simulink model "estymacja_obiekt2_18a"  (R2018a)
settings: Solver=FixedStepDiscrete  StartTime=0.0  StopTime=10.0  FixedStep=0.1  RelTol=1e-3
libraries: sharedTrackingLibrary x1
settings Model: Creator=Dominik  LastModifiedBy=a.kuligowski
settings CodeAppCC: StateflowObjectComments=on

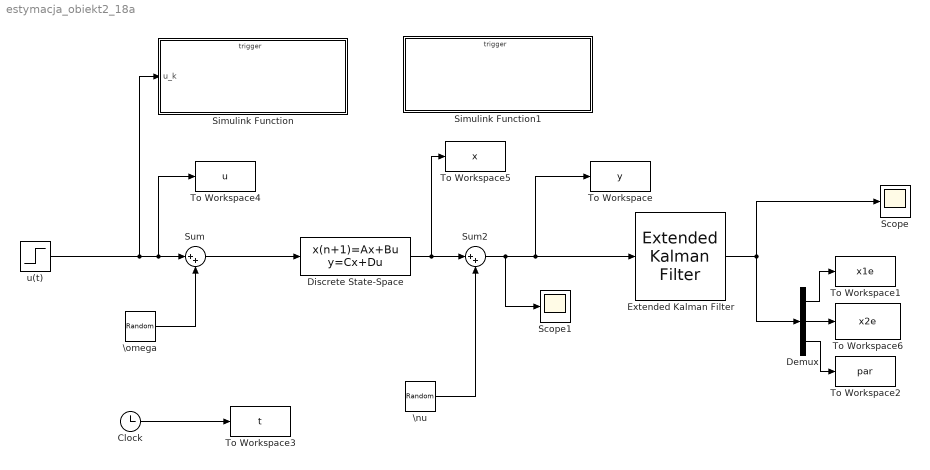
== system estymacja_obiekt2_18a ==
  Clock : Clock
  Demux : Demux  Outputs=3
  Discrete State-Space : DiscreteStateSpace  A=[0.99 0.095; -0.19 0.9]  B=[0.005; 0.095]  C=[1 0]  D=0  InitialCondition=[0;0]  SampleTime=0.1
  Extended Kalman Filter : sharedTrackingLibrary/Extended Kalman Filter  StateTransitionFcn=myStateTransitionFcn  HasStateTransitionJacobianFcn=off  HasAdditiveProcessNoise=Additive  ProcessNoise=diag([0.0005 0.0005 0.0005])  HasTimeVaryingProcessNoise=off  HasStateTransitionFcnExtraArgument=0  InitialState=[0 0 0.2]  InitialStateCovariance=1  MeasurementFcn1=myMeasurementFcn  HasMeasurementJacobianFcn1=off  HasMeasurementEnablePort1=off  HasAdditiveMeasurementNoise1=Additive  MeasurementNoise1=0.0001  HasTimeVaryingMeasurementNoise1=off  HasMeasurementFcnExtraArgument1=0  MeasurementFcn2=myMeasurementFcn  HasMeasurementJacobianFcn2=off  HasMeasurementEnablePort2=off  HasAdditiveMeasurementNoise2=Additive  MeasurementNoise2=1  HasTimeVaryingMeasurementNoise2=off  HasMeasurementFcnExtraArgument2=0  MeasurementFcn3=myMeasurementFcn  HasMeasurementJacobianFcn3=off  HasMeasurementEnablePort3=off  HasAdditiveMeasurementNoise3=Additive  MeasurementNoise3=1  HasTimeVaryingMeasurementNoise3=off  HasMeasurementFcnExtraArgument3=0  MeasurementFcn4=myMeasurementFcn  HasMeasurementJacobianFcn4=off  HasMeasurementEnablePort4=off  HasAdditiveMeasurementNoise4=Additive  MeasurementNoise4=1  HasTimeVaryingMeasurementNoise4=off  HasMeasurementFcnExtraArgument4=0  MeasurementFcn5=myMeasurementFcn  HasMeasurementJacobianFcn5=off  HasMeasurementEnablePort5=off  HasAdditiveMeasurementNoise5=Additive  MeasurementNoise5=1  HasTimeVaryingMeasurementNoise5=off  HasMeasurementFcnExtraArgument5=0  EnableMultirate=off  StateTransitionFcnSampleTime=1  MeasurementFcn1SampleTime=1  MeasurementFcn2SampleTime=1  MeasurementFcn3SampleTime=1  MeasurementFcn4SampleTime=1  MeasurementFcn5SampleTime=1  UseCurrentEstimator=on  OutputStateCovariance=off  DataType=double  SampleTime=0.1  NumberOfMeasurements=1
      settings: SourceProductName=Control System Toolbox  SourceProductBaseCode=CT
  Scope : Scope
  Scope1 : Scope
  Simulink Function : Subsystem  TreatAsAtomicUnit=on
  Simulink Function1 : Subsystem  TreatAsAtomicUnit=on
  Sum : Sum  Inputs=|++
  Sum2 : Sum  Inputs=|++
  To Workspace : ToWorkspace  VariableName=y  SampleTime=-1
  To Workspace1 : ToWorkspace  VariableName=x1e  SampleTime=-1
  To Workspace2 : ToWorkspace  VariableName=par  SampleTime=-1
  To Workspace3 : ToWorkspace  VariableName=t  SampleTime=-1
  To Workspace4 : ToWorkspace  VariableName=u  SampleTime=-1
  To Workspace5 : ToWorkspace  VariableName=x  SampleTime=-1
  To Workspace6 : ToWorkspace  VariableName=x2e  SampleTime=-1
  \nu : RandomNumber  Variance=0  Seed=11  SampleTime=0.1
  \omega : RandomNumber  Variance=0.0005  Seed=21  SampleTime=0.1
  u(t) : Step  SampleTime=0
  wires:
  Extended Kalman Filter/1 -> Demux/1, Scope/1
  Discrete State-Space/1 -> To Workspace5/1, Sum2/1
  Sum2/1 -> Scope1/1, To Workspace/1, Extended Kalman Filter/1
  \omega/1 -> Sum/2
  \nu/1 -> Sum2/2
  u(t)/1 -> Simulink Function/1(u_k), To Workspace4/1, Sum/1
  Demux/3 -> To Workspace2/1
  Demux/1 -> To Workspace1/1
  Clock/1 -> To Workspace3/1
  Sum/1 -> Discrete State-Space/1
  Demux/2 -> To Workspace6/1

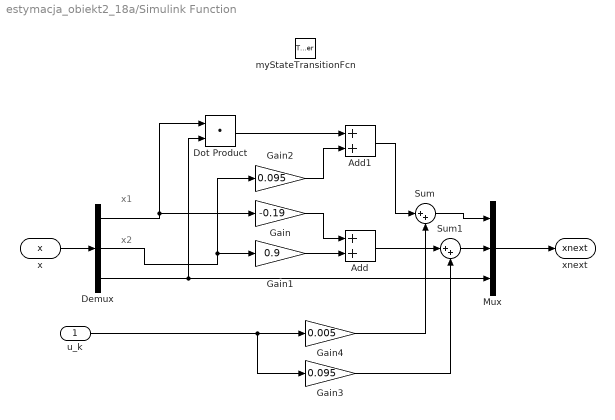
== system estymacja_obiekt2_18a/Simulink Function ==
  note: x2
  note: x1
  u_k : Inport
  myStateTransitionFcn : TriggerPort  TriggerType=function-call  IsSimulinkFunction=on  FunctionName=myStateTransitionFcn  VariantControl=Variant
  Add : Sum
  Add1 : Sum
  Demux : Demux  Outputs=3
  Dot Product : DotProduct  InputSameDT=on  OutDataTypeStr=Inherit: Inherit via internal rule
  Gain : Gain  Gain=-0.19
  Gain1 : Gain  Gain=0.9
  Gain2 : Gain  Gain=0.095
  Gain3 : Gain  Gain=0.095
  Gain4 : Gain  Gain=0.005
  Mux : Mux  Inputs=3
  Sum : Sum  Inputs=|++
  Sum1 : Sum  Inputs=|++
  x : ArgIn  DisableCoverage=on  PortDimensions=3  ArgumentName=x
  xnext : ArgOut  DisableCoverage=on  PortDimensions=3  ArgumentName=xnext
  wires:
  x/1 -> Demux/1
  Demux/3 -> Mux/3, Dot Product/2
  Dot Product/1 -> Add1/1
  Demux/1 -> Dot Product/1, Gain/1
  Sum/1 -> Mux/1
  Mux/1 -> xnext/1
  u_k/1 -> Gain3/1, Gain4/1
  Demux/2 -> Gain2/1, Gain1/1
  Gain4/1 -> Sum/2
  Sum1/1 -> Mux/2
  Gain3/1 -> Sum1/2
  Add/1 -> Sum1/1
  Gain/1 -> Add/1
  Gain1/1 -> Add/2
  Add1/1 -> Sum/1
  Gain2/1 -> Add1/2

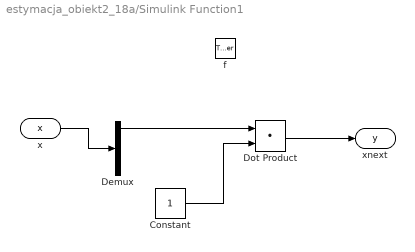
== system estymacja_obiekt2_18a/Simulink Function1 ==
  f : TriggerPort  TriggerType=function-call  IsSimulinkFunction=on  FunctionName=myMeasurementFcn  VariantControl=Variant
  Constant : Constant
  Demux : Demux  Outputs=3
  Dot Product : DotProduct  InputSameDT=on  OutDataTypeStr=Inherit: Inherit via internal rule
  x : ArgIn  DisableCoverage=on  PortDimensions=3  ArgumentName=x
  xnext : ArgOut  DisableCoverage=on  ArgumentName=y
  wires:
  Dot Product/1 -> xnext/1
  Constant/1 -> Dot Product/2
  x/1 -> Demux/1
  Demux/1 -> Dot Product/1
